simulink model "the_system"  (R2023a)
settings: Solver=ode3  StartTime=0.0  StopTime=10.0  FixedStep=0.002  RelTol=1e-3
libraries: simulink x1
settings Model: Creator=ElvisJu  LastModifiedBy=ElvisJu

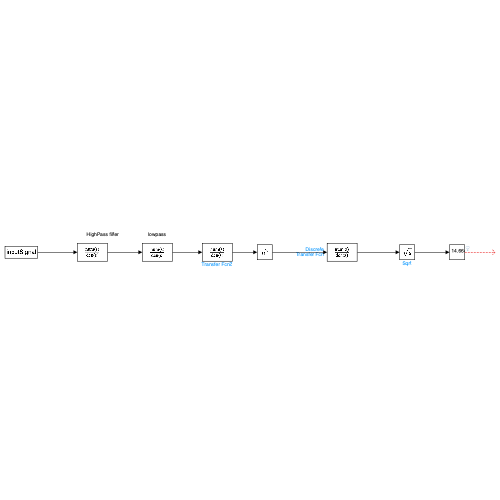
[thumbnail: Simulink's stored preview of the top-level diagram]
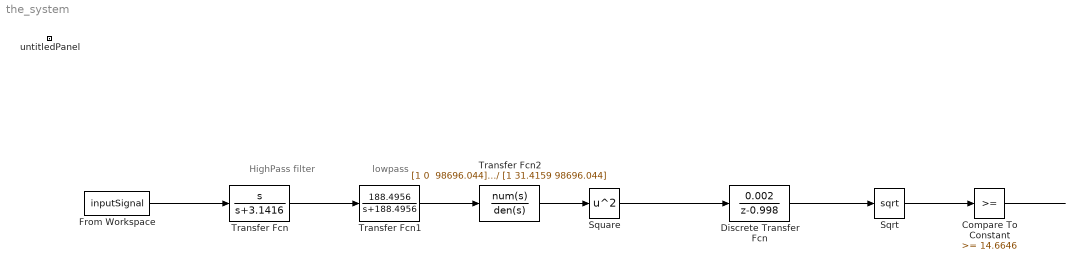
== system the_system ==
  note: lowpass
  note: HighPass filter
  Compare To Constant : simulink/Logic and Bit Operations/Compare To Constant  relop=>=  const=14.6646  OutDataTypeStr=boolean
  Discrete Transfer Fcn : DiscreteTransferFcn  Numerator=[0.002]  Denominator=[1 -0.998]  SampleTime=0.002
  From Workspace : FromWorkspace  VariableName=inputSignal  SampleTime=0.002  OutputAfterFinalValue=Setting to zero
  Sqrt : Sqrt
  Square : Math  Operator=square
  Transfer Fcn : TransferFcn  Numerator=[1 0]  Denominator=[1 3.1416]
  Transfer Fcn1 : TransferFcn  Numerator=[188.4956]  Denominator=[1 188.4956]
  Transfer Fcn2 : TransferFcn  Numerator="[1 0  98696.044]"  Denominator=[1 31.4159 98696.044]
  untitledPanel : Subsystem  Tag=HiddenForWebPanel  IsWebBlockPanel=on
  wires:
  From Workspace/1 -> Transfer Fcn/1
  Transfer Fcn2/1 -> Square/1
  Sqrt/1 -> Compare To Constant/1
  Square/1 -> Discrete Transfer Fcn/1
  Transfer Fcn/1 -> Transfer Fcn1/1
  Transfer Fcn1/1 -> Transfer Fcn2/1
  Discrete Transfer Fcn/1 -> Sqrt/1
  Compare To Constant/1 -> ?

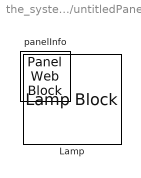
== system the_system/untitledPanel ==
  Lamp : LampBlock  Tag=HiddenForWebPanel  PanelInfo="{\"height\":90,\"left\":18,\"panelId\":\"panelId-48913d2b-f7e8-4c19-976f-3532a2d7365c\",\"top\":18,\"type\":\"panelChild\",\"version\":\"2019b\",\"width\":98,\"zIndex\":1499998}"  LabelPosition=Bottom
  panelInfo : PanelWebBlock  Tag=HiddenForWebPanel  PanelInfo="{\"compacted\":false,\"height\":130,\"isActiveTab\":true,\"left\":894,\"name\":\"Panel\",\"panelId\":\"panelId-48913d2b-f7e8-4c19-976f-3532a2d7365c\",\"tabIndex\":0,\"tabbedSetId\":\"tabbedSet9113335984\",\"top\":198,\"type\":\"panel\",\"version\":\"2019b\",\"visible\":true,\"width\":138,\"zIndex\":1500002}"
